simulink model "mekf_nocontrol_test"  (R2018b)
settings: Solver=VariableStepAuto  StartTime=0.0  StopTime=5600  RelTol=1e-3
undefined symbols (not defined in the file or in its folder): fswParams, mtq_dipole_body_Am2, rwa_torque_body_Nm
libraries: Environment_lib x1, MEKF_lib x1, actuator_control_bus x1, quat_err_lib x1, satelliteDynamics_lib x1, aerolibutil x1, gyroscope_lib x1, magnetometer_lib x1
settings Model: Creator=Taylor  LastModifiedBy=Taylor

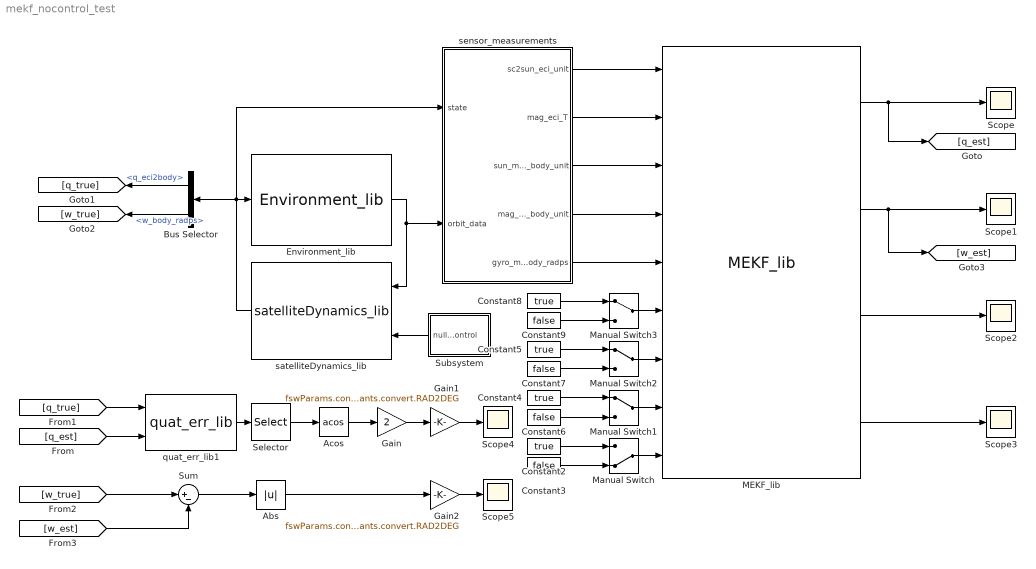
== system mekf_nocontrol_test ==
  Abs : Abs
  Acos : Trigonometry  Operator=acos
  Bus Selector : BusSelector  OutputSignals=q_eci2body,w_body_radps
  Constant{2,4..5,8} (4 alike) : Constant  Value=true
  Constant{3,6..7,9} (4 alike) : Constant  Value=false
  Environment_lib : Environment_lib/Environment_lib  SystemSampleTime=-1
  Gain : Gain  Gain=2
  Gain1 : Gain  Gain=fswParams.constants.convert.RAD2DEG
  Gain2 : Gain  Gain=fswParams.constants.convert.RAD2DEG
  MEKF_lib : MEKF_lib/MEKF_lib  SystemSampleTime=-1
  Manual Switch : ManualSwitch  CurrentSetting=0
  Manual Switch1 : ManualSwitch
  Manual Switch2 : ManualSwitch
  Manual Switch3 : ManualSwitch
  Scope{,1..5} (6 alike) : Scope
  Selector : Selector  InputPortWidth=4  IndexOptions=Index vector (dialog)  Indices=[1]  OutputSizes=1
  Subsystem : Subsystem
  Sum : Sum  Inputs=|+-
  quat_err_lib1 : quat_err_lib/quat_err_lib  SystemSampleTime=-1
  satelliteDynamics_lib : satelliteDynamics_lib/satelliteDynamics_lib  SystemSampleTime=-1
  sensor_measurements : Subsystem
  wires:
  satelliteDynamics_lib/1 -> Bus Selector/1, sensor_measurements/1(state), Environment_lib/1
  Environment_lib/1 -> sensor_measurements/2(orbit_data), satelliteDynamics_lib/1
  Constant7/1 -> Manual Switch2/2
  Constant4/1 -> Manual Switch1/1
  Constant6/1 -> Manual Switch1/2
  Constant5/1 -> Manual Switch2/1
  Constant2/1 -> Manual Switch/1
  Constant9/1 -> Manual Switch3/2
  Constant3/1 -> Manual Switch/2
  Manual Switch3/1 -> MEKF_lib/6
  Manual Switch/1 -> MEKF_lib/9
  Manual Switch1/1 -> MEKF_lib/8
  Manual Switch2/1 -> MEKF_lib/7
  Constant8/1 -> Manual Switch3/1
  Subsystem/1(null_control) -> satelliteDynamics_lib/2
  MEKF_lib/1 -> [q_est], Scope/1
  MEKF_lib/2 -> [w_est], Scope1/1
  MEKF_lib/3 -> Scope2/1
  MEKF_lib/4 -> Scope3/1
  sensor_measurements/5(gyro_meas_body_radps) -> MEKF_lib/5
  sensor_measurements/4(mag_meas_body_unit) -> MEKF_lib/4
  sensor_measurements/3(sun_meas_body_unit) -> MEKF_lib/3
  sensor_measurements/2(mag_eci_T) -> MEKF_lib/2
  sensor_measurements/1(sc2sun_eci_unit) -> MEKF_lib/1
  Bus Selector/1 -> [q_true]  "<q_eci2body>"
  [q_true] -> quat_err_lib1/1
  [q_est] -> quat_err_lib1/2
  Selector/1 -> Acos/1
  Gain1/1 -> Scope4/1
  Acos/1 -> Gain/1
  Gain/1 -> Gain1/1
  quat_err_lib1/1 -> Selector/1
  Bus Selector/2 -> [w_true]  "<w_body_radps>"
  [w_true] -> Sum/1
  [w_est] -> Sum/2
  Sum/1 -> Abs/1
  Abs/1 -> Gain2/1
  Gain2/1 -> Scope5/1

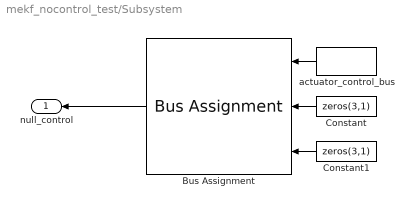
== system mekf_nocontrol_test/Subsystem ==
  Bus Assignment : BusAssignment  AssignedSignals=rwa_torque_body_Nm,mtq_dipole_body_Am2
  Constant : Constant  Value=zeros(3,1)
  Constant1 : Constant  Value=zeros(3,1)
  actuator_control_bus : actuator_control_bus/actuator_control_bus  SystemSampleTime=-1
  null_control : Outport
  wires:
  Bus Assignment/1 -> null_control/1
  Constant1/1 -> Bus Assignment/3
  Constant/1 -> Bus Assignment/2
  actuator_control_bus/1 -> Bus Assignment/1

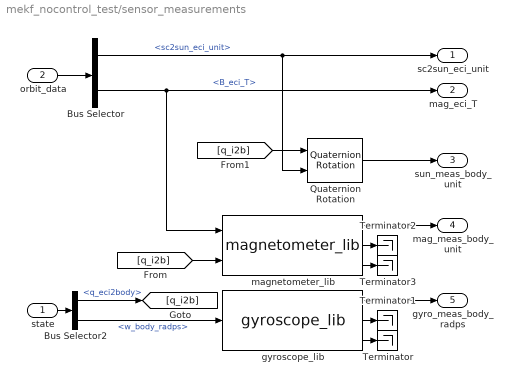
== system mekf_nocontrol_test/sensor_measurements ==
  state : Inport
  orbit_data : Inport  Port=2
  Bus Selector : BusSelector  OutputSignals=sc2sun_eci_unit,B_eci_T
  Bus Selector2 : BusSelector  OutputSignals=q_eci2body,w_body_radps
  Quaternion Rotation : aerolibutil/Quaternion Rotation
  Terminator{,1..3} (4 alike) : Terminator
  gyroscope_lib : gyroscope_lib/gyroscope_lib  id_s=1
  magnetometer_lib : magnetometer_lib/magnetometer_lib  id_s=1
  sc2sun_eci_unit : Outport
  mag_eci_T : Outport  Port=2
  sun_meas_body_unit : Outport  Port=3
  mag_meas_body_unit : Outport  Port=4
  gyro_meas_body_radps : Outport  Port=5
  wires:
  state/1 -> Bus Selector2/1
  orbit_data/1 -> Bus Selector/1
  Quaternion Rotation/1 -> sun_meas_body_unit/1
  magnetometer_lib/1 -> mag_meas_body_unit/1
  gyroscope_lib/1 -> gyro_meas_body_radps/1
  gyroscope_lib/3 -> Terminator/1
  gyroscope_lib/2 -> Terminator1/1
  Bus Selector2/2 -> gyroscope_lib/1  "<w_body_radps>"
  Bus Selector2/1 -> [q_i2b]  "<q_eci2body>"
  magnetometer_lib/2 -> Terminator2/1
  magnetometer_lib/3 -> Terminator3/1
  [q_i2b] -> magnetometer_lib/2
  [q_i2b] -> Quaternion Rotation/1
  Bus Selector/2 -> magnetometer_lib/1, mag_eci_T/1  "<B_eci_T>"
  Bus Selector/1 -> Quaternion Rotation/2, sc2sun_eci_unit/1  "<sc2sun_eci_unit>"
